simulink model "sfcndemo_sfun_zc_sat"  (Simulink 7.6)
settings: Solver=VariableStepDiscrete  SolverMode=SingleTasking  StartTime=0.0  StopTime=10.0  RelTol=1e-3
Description:
  | Saturation Using Non-Sampled Zero Crossings C-MEX S-function
settings Model: Creator=The MathWorks Inc.  ExtModeTrigMode=oneshot  ExtModeArmWhenConnect=off  ExtModeAutoUpdateStatusClock=off
settings DataIOCC: LimitDataPoints=off
settings OptimizationCC: BlockReduction=off  BooleanDataType=off  InitFltsAndDblsToZero=on
settings DebuggingCC: SaveWithParameterizedLinksMsg=none  SignalResolutionControl=TryResolveAllWithWarning  SolverPrmCheckMsg=none  InheritedTsInSrcMsg=none  MultiTaskDSMMsg=warning  MultiTaskCondExecSysMsg=none
settings HardwareCC: TargetUnknown=on
settings RTWCC: IncludeERTFirstTime=on
settings CodeAppCC: CustomSymbolStrFcn=$F$N$M
settings GRTTargetCC: TargetFcnLib=ansi_tfl_tmw.mat

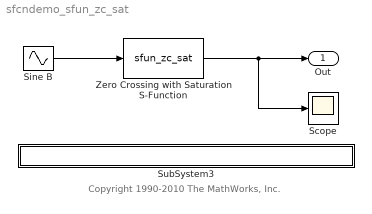
== system sfcndemo_sfun_zc_sat ==
  note: Copyright 1990-2010 The MathWorks, Inc.
  Scope : Scope
      settings: TimeRange=10  YMin=-0.5  YMax=1  SampleInput=on
  Sine B : Sin
  SubSystem3 : Subsystem  mask{filename=sfun_zc_sat.c}
      mask init:
      | x=sfundemo_maskdisp;
      settings: AttributesFormatString=\n  OpenFcn=sfundemo_openfcn
      mask Display: disp(x);
  Zero Crossing with Saturation S-Function : S-Function  FunctionName=sfun_zc_sat  Parameters=ub, lb  EnableBusSupport=off  mask(S-function: sfun_zc_sat){ub=[0.5 0.75], lb=[0,-.5]}
      mask prompts: ub "Upper Limit"; lb "Lower Limit"
      mask help: This is a S-function block which has nonsampled zero crossings to implement a saturation function.
  Out : Outport  InitialOutput=0
  wires:
  Sine B/1 -> Zero Crossing with Saturation S-Function/1
  Zero Crossing with Saturation S-Function/1 -> Out/1, Scope/1

== system sfcndemo_sfun_zc_sat/SubSystem3 ==
